simulink model "Copy_of_sliding_controller"  (R2021a)
settings: Solver=FixedStepAuto  StartTime=0.0  StopTime=inf  FixedStep=0.02  RelTol=1e-3
model workspace (MAT data in the model file):
  SL_ROS_VariableLengthArrays_MaxSizes.CommonInfo.ArrayTruncateAction = 'EmitWarning'
  SL_ROS_VariableLengthArrays_MaxSizes.MsgTypeMap = containers.Map
  SL_ROS_VariableLengthArrays_MaxSizes.MsgTypeMap.serialization.keys = {'ambf_walker/DesiredJoints', 'rbdl_server/RBDLInverseDynamicsRequest', 'rbdl_server/RBDLInverseDynamicsResponse', 'sensor_msgs/JointState'}
  SL_ROS_VariableLengthArrays_MaxSizes.MsgTypeMap.serialization.values{1}(1).PropertyName = 'Controller'
  SL_ROS_VariableLengthArrays_MaxSizes.MsgTypeMap.serialization.values{1}(1).DataType = 'uint8'
  SL_ROS_VariableLengthArrays_MaxSizes.MsgTypeMap.serialization.values{1}(1).MaxLength = 8
  SL_ROS_VariableLengthArrays_MaxSizes.MsgTypeMap.serialization.values{1}(2).PropertyName = 'Other'
  SL_ROS_VariableLengthArrays_MaxSizes.MsgTypeMap.serialization.values{1}(2).DataType = 'double'
  SL_ROS_VariableLengthArrays_MaxSizes.MsgTypeMap.serialization.values{1}(2).MaxLength = 7
  SL_ROS_VariableLengthArrays_MaxSizes.MsgTypeMap.serialization.values{1}(3).PropertyName = 'Q'
  SL_ROS_VariableLengthArrays_MaxSizes.MsgTypeMap.serialization.values{1}(3).DataType = 'double'
  SL_ROS_VariableLengthArrays_MaxSizes.MsgTypeMap.serialization.values{1}(3).MaxLength = 7
  SL_ROS_VariableLengthArrays_MaxSizes.MsgTypeMap.serialization.values{1}(4).PropertyName = 'Qd'
  SL_ROS_VariableLengthArrays_MaxSizes.MsgTypeMap.serialization.values{1}(4).DataType = 'double'
  SL_ROS_VariableLengthArrays_MaxSizes.MsgTypeMap.serialization.values{1}(4).MaxLength = 7
  SL_ROS_VariableLengthArrays_MaxSizes.MsgTypeMap.serialization.values{1}(5).PropertyName = 'Qdd'
  SL_ROS_VariableLengthArrays_MaxSizes.MsgTypeMap.serialization.values{1}(5).DataType = 'double'
  SL_ROS_VariableLengthArrays_MaxSizes.MsgTypeMap.serialization.values{1}(5).MaxLength = 7
  SL_ROS_VariableLengthArrays_MaxSizes.MsgTypeMap.serialization.values{2}(1).PropertyName = 'ModelName'
  SL_ROS_VariableLengthArrays_MaxSizes.MsgTypeMap.serialization.values{2}(1).DataType = 'uint8'
  SL_ROS_VariableLengthArrays_MaxSizes.MsgTypeMap.serialization.values{2}(1).MaxLength = 31
  SL_ROS_VariableLengthArrays_MaxSizes.MsgTypeMap.serialization.values{2}(2).PropertyName = 'Q'
  SL_ROS_VariableLengthArrays_MaxSizes.MsgTypeMap.serialization.values{2}(2).DataType = 'double'
  SL_ROS_VariableLengthArrays_MaxSizes.MsgTypeMap.serialization.values{2}(2).MaxLength = 7
  SL_ROS_VariableLengthArrays_MaxSizes.MsgTypeMap.serialization.values{2}(3).PropertyName = 'Qd'
  SL_ROS_VariableLengthArrays_MaxSizes.MsgTypeMap.serialization.values{2}(3).DataType = 'double'
  SL_ROS_VariableLengthArrays_MaxSizes.MsgTypeMap.serialization.values{2}(3).MaxLength = 7
  SL_ROS_VariableLengthArrays_MaxSizes.MsgTypeMap.serialization.values{2}(4).PropertyName = 'Qdd'
  SL_ROS_VariableLengthArrays_MaxSizes.MsgTypeMap.serialization.values{2}(4).DataType = 'double'
  SL_ROS_VariableLengthArrays_MaxSizes.MsgTypeMap.serialization.values{2}(4).MaxLength = 7
  SL_ROS_VariableLengthArrays_MaxSizes.MsgTypeMap.serialization.values{3}.PropertyName = 'Tau'
  SL_ROS_VariableLengthArrays_MaxSizes.MsgTypeMap.serialization.values{3}.DataType = 'double'
  SL_ROS_VariableLengthArrays_MaxSizes.MsgTypeMap.serialization.values{3}.MaxLength = 7
  SL_ROS_VariableLengthArrays_MaxSizes.MsgTypeMap.serialization.values{4}(1).PropertyName = 'Effort'
  SL_ROS_VariableLengthArrays_MaxSizes.MsgTypeMap.serialization.values{4}(1).DataType = 'double'
  SL_ROS_VariableLengthArrays_MaxSizes.MsgTypeMap.serialization.values{4}(1).MaxLength = 7
  SL_ROS_VariableLengthArrays_MaxSizes.MsgTypeMap.serialization.values{4}(2).PropertyName = 'Name'
  SL_ROS_VariableLengthArrays_MaxSizes.MsgTypeMap.serialization.values{4}(2).DataType = 'std_msgs/String'
  SL_ROS_VariableLengthArrays_MaxSizes.MsgTypeMap.serialization.values{4}(2).MaxLength = 16
  SL_ROS_VariableLengthArrays_MaxSizes.MsgTypeMap.serialization.values{4}(3).PropertyName = 'Position'
  SL_ROS_VariableLengthArrays_MaxSizes.MsgTypeMap.serialization.values{4}(3).DataType = 'double'
  SL_ROS_VariableLengthArrays_MaxSizes.MsgTypeMap.serialization.values{4}(3).MaxLength = 7
  SL_ROS_VariableLengthArrays_MaxSizes.MsgTypeMap.serialization.values{4}(4).PropertyName = 'Velocity'
  SL_ROS_VariableLengthArrays_MaxSizes.MsgTypeMap.serialization.values{4}(4).DataType = 'double'
  SL_ROS_VariableLengthArrays_MaxSizes.MsgTypeMap.serialization.values{4}(4).MaxLength = 7
  SL_ROS_VariableLengthArrays_MaxSizes.MsgTypeMap.serialization.uniformity = 0
  SL_ROS_VariableLengthArrays_MaxSizes.MsgTypeMap.serialization.keyType = 'char'
  SL_ROS_VariableLengthArrays_MaxSizes.MsgTypeMap.serialization.valueType = 'any'
values from neighbouring files (symbols this model uses):
  dampener = [30, 0; 0, 30]    [init_with_opt_gains.m]    (also in sliding_controller_init.m = 100*eye(2); trying01.m; trying02.m = [0.30, 0; 0, 0.30])
  Dm1 = [Dm_hip, 0.0, 0.0, 0.0, 0.0, 0.0,0 ... (first row only)    [init_with_opt_gains.m]    (also in sliding_controller_init.m = 30*eye(7); trying01.m; trying02.m = [101.7013888888889 0 0 0 0 0)
  exo_sat = 50    [init_with_opt_gains.m]    (also in sliding_controller_init.m; trying01.m = 250; trying02.m = 30)
  invMd = inv(Md)    [init_with_opt_gains.m]    (also in sliding_controller_init.m; trying01.m; trying02.m)
  Km1 = [Km_hip, 0.0, 0.0, 0.0, 0.0, 0.0,0 ... (first row only)    [init_with_opt_gains.m]    (also in sliding_controller_init.m = 30*eye(7); trying01.m; trying02.m = [6120.116528948097 0 0 0 0 0)
  l = [ 1.0, 1.5]    [sliding_controller_init.m]
  lambda2 = [lambda_hip, 0, 0, 0, 0, 0,0 ... (first row only)    [init_with_opt_gains.m]    (also in sliding_controller_init.m = eye(7); trying01.m; trying02.m = [lambda_hip, 0, 0, 0, 0, 0)
  mh = [2, 1]    [sliding_controller_init.m]
  rho2 = [rho_hip, 0.0, 0.0, 0.0, 0.0, 0.0,0 ... (first row only)    [init_with_opt_gains.m]    (also in sliding_controller_init.m = 200*eye(7); trying01.m; trying02.m = [rho_hip, 0.0, 0.0, 0.0, 0.0, 0.0)
  sat = 10    [sliding_controller_init.m]
  spring = [30, 0; 0, 30]    [init_with_opt_gains.m]    (also in sliding_controller_init.m = 100*eye(2); trying01.m; trying02.m = [0.30, 0; 0, 0.30])
undefined symbols (not defined in the file or in its folder): ModelName, Q, Qd, Qdd
libraries: robotlib x14
settings Model: Creator=nathanielgoldfarb  LastModifiedBy=nathanielgoldfarb
settings OptimizationCC: DefaultParameterBehavior=Inlined  EnhancedBackFolding=on  PassReuseOutputArgsAs=Individual arguments  ZeroExternalMemoryAtStartup=off  ZeroInternalMemoryAtStartup=off  InitFltsAndDblsToZero=on  MaxStackSize=64  OptimizeBlockOrder=speed  DifferentSizesBufferReuse=on  OptimizationCustomize=off  EfficientTunableParamExpr=on
settings DebuggingCC: ParameterTunabilityLossMsg=error
settings HardwareCC: TargetLongLongMode=on  UseEmbeddedCoderFeatures=off
settings SFSimCC: MATLABDynamicMemAlloc=off
settings RTWCC: SystemTargetFile=ert.tlc  TemplateMakefile=ert_default_tmf  Toolchain=Catkin
settings CodeAppCC: ForceParamTrailComments=on  IgnoreCustomStorageClasses=off  OperatorAnnotations=on  SimulinkDataObjDesc=on  SFDataObjDesc=on  InsertBlockDesc=on
settings ERTTargetCC: GenerateSampleERTMain=on  InlinedParameterPlacement=NonHierarchical  ERTCustomFileTemplate=example_file_process.tlc

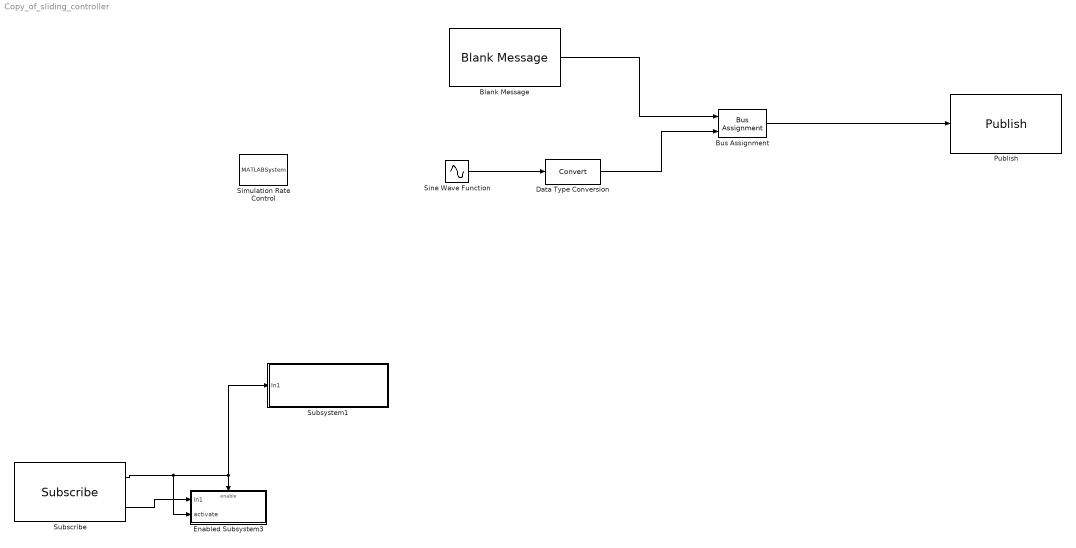
== system Copy_of_sliding_controller ==
  Blank Message : robotlib/Blank Message  messageClass=Message  entityType=std_msgs/Float32  messageType=std_msgs/Float32  SampleTime=-1  legacyBusStruct=off
  Bus Assignment : BusAssignment  AssignedSignals=Data
  Data Type Conversion : DataTypeConversion
  Enabled Subsystem3 : Subsystem  TreatAsAtomicUnit=on
  Publish : robotlib/Publish  topicSource=Specify your own  topic=/sin_wave  messageType=std_msgs/Float32  legacyBusStruct=off  messageQueueLength=1
  Simulation Rate Control : MATLABSystem  System=ExampleHelperSimulationRateControl  SampleTime=.02
      mask Type: ExampleHelperSimulationRateControl
      mask Display: disp('Rate Control');
  Sine Wave Function : Sin  SampleTime=0
  Subscribe : robotlib/Subscribe  topicSource=Select from ROS network  topic=/exosimulink_set_points  messageType=ambf_walker/DesiredJoints  SampleTime=-1  legacyBusStruct=off  messageQueueLength=1
  Subsystem1 : Subsystem
  wires:
  Subscribe/1 -> Enabled Subsystem3/2(activate), Subsystem1/1(In1), Enabled Subsystem3/Enable
  Data Type Conversion/1 -> Bus Assignment/2
  Blank Message/1 -> Bus Assignment/1
  Sine Wave Function/1 -> Data Type Conversion/1
  Bus Assignment/1 -> Publish/1
  Subscribe/2 -> Enabled Subsystem3/1(In1)

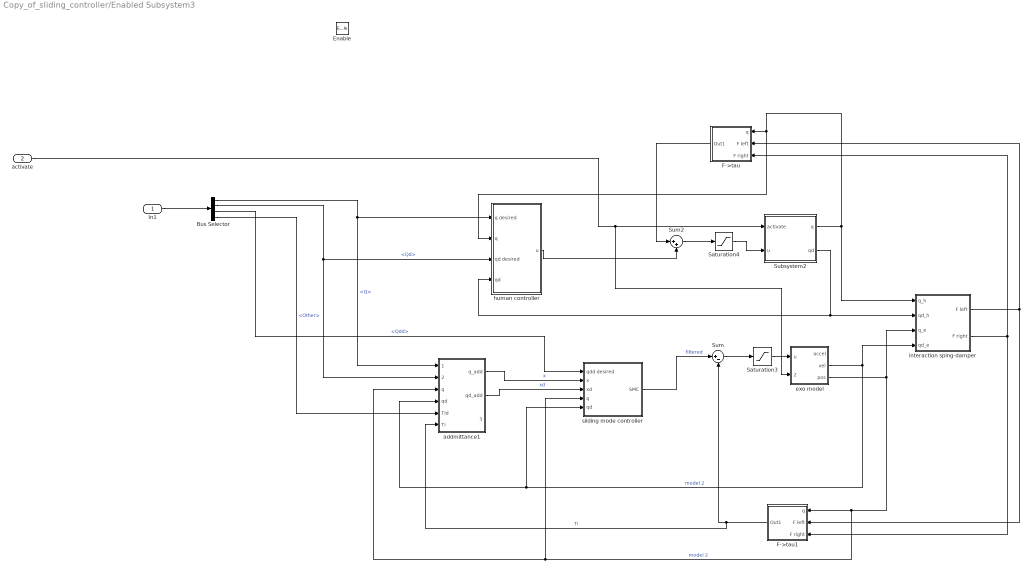
== system Copy_of_sliding_controller/Enabled Subsystem3 ==
  In1 : Inport
  activate : Inport  Port=2
  Enable : EnablePort
  " interaction sping-damper" : Subsystem
  Bus Selector : BusSelector  OutputSignals=Q,Qd,Qdd,Other
  F->tau : Subsystem
  F->tau1 : Subsystem
  Saturation3 : Saturate  UpperLimit=exo_sat  LowerLimit=-exo_sat
  Saturation4 : Saturate  UpperLimit=exo_sat  LowerLimit=-exo_sat
  Subsystem2 : Subsystem
  Sum : Sum  Inputs=|+-
  Sum2 : Sum  Inputs=|++
  addmittance1 : Subsystem
  exo model : Subsystem
  human controller : Subsystem
  sliding mode controller : Subsystem
  wires:
  exo model/3(pos) -> " interaction sping-damper"/3(q_e), addmittance1/3(q), sliding mode controller/4(q), F->tau1/1(q)  "model 2"
  Bus Selector/4 -> addmittance1/5(Tid)  "<Other>"
  Saturation3/1 -> exo model/1(u)
  addmittance1/2(qd_add) -> sliding mode controller/3(xd)  "xd"
  exo model/2(vel) -> " interaction sping-damper"/4("qd_e "), addmittance1/4(qd), sliding mode controller/5(qd)  "model 2"
  sliding mode controller/1(SMC) -> Sum/1  "filtered"
  " interaction sping-damper"/2(F right) -> F->tau1/3(F right), F->tau/3(F right)
  In1/1 -> Bus Selector/1
  human controller/1(u) -> Sum2/2
  Bus Selector/1 -> addmittance1/1(q desird), human controller/1(q desired)  "<Q>"
  Subsystem2/1(q) -> F->tau/1(q), human controller/2(q), " interaction sping-damper"/1(q_h)
  " interaction sping-damper"/1(F left) -> F->tau1/2(F left), F->tau/2(F left)
  Saturation4/1 -> Subsystem2/2(u)
  F->tau/1(Out1) -> Sum2/1
  addmittance1/1(q_add) -> sliding mode controller/2(x)  "x"
  Bus Selector/3 -> sliding mode controller/1(qdd desired)  "<Qdd>"
  Sum/1 -> Saturation3/1
  Bus Selector/2 -> addmittance1/2(qd desird), human controller/3(qd desired)  "<Qd>"
  Sum2/1 -> Saturation4/1
  Subsystem2/2(qd) -> human controller/4(qd), " interaction sping-damper"/2(qd_h)
  F->tau1/1(Out1) -> Sum/2, addmittance1/6(Ti)  "Ti"
  activate/1 -> exo model/2(activate), Subsystem2/1(activate)

== system Copy_of_sliding_controller/Subsystem1 ==
  In1 : Inport
  Constant : Constant  Value=false
  Data Type Conversion : DataTypeConversion
  If : If  IfExpression=u1 == 1
  If Action Subsystem : Subsystem  TreatAsAtomicUnit=on
  wires:
  In1/1 -> Data Type Conversion/1
  If/1 -> If Action Subsystem/Action
  Data Type Conversion/1 -> If/1
  Constant/1 -> If Action Subsystem/1(In1)

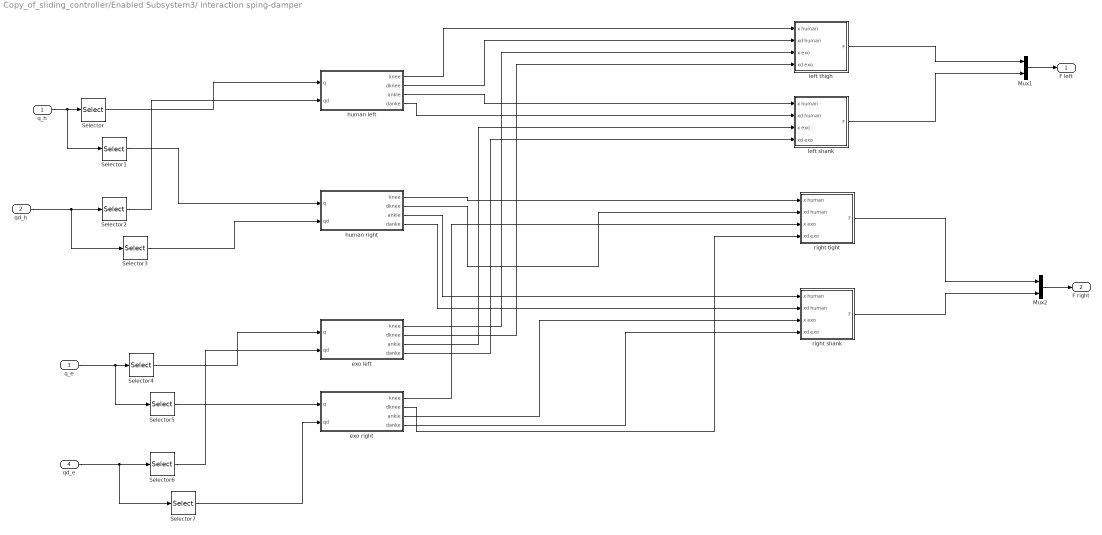
== system Copy_of_sliding_controller/Enabled Subsystem3/ interaction sping-damper ==
  q_h : Inport
  qd_h : Inport  Port=2
  q_e : Inport  Port=3
  "qd_e " : Inport  Port=4
  Mux1 : Mux  Inputs=2
  Mux2 : Mux  Inputs=2
  Selector{,2,4,6} (4 alike) : Selector  InputPortWidth=7  IndexOptions=Index vector (dialog)  Indices=[1 2]  OutputSizes=1
  Selector{1,3,5,7} (4 alike) : Selector  InputPortWidth=7  IndexOptions=Index vector (dialog)  Indices=[4 5]  OutputSizes=1
  exo left : MATLAB Function  TreatAsAtomicUnit=on
  exo right : MATLAB Function  TreatAsAtomicUnit=on
  human left : MATLAB Function  TreatAsAtomicUnit=on
  human right : MATLAB Function  TreatAsAtomicUnit=on
  left shank : Subsystem
  left thigh : Subsystem
  right shank : Subsystem
  right tight : Subsystem
  F left : Outport
  F right : Outport  Port=2
  wires:
  q_h/1 -> Selector1/1, Selector/1
  Selector/1 -> human left/1(q)
  Selector1/1 -> human right/1(q)
  Selector2/1 -> human left/2(qd)
  Selector3/1 -> human right/2(qd)
  qd_h/1 -> Selector3/1, Selector2/1
  q_e/1 -> Selector5/1, Selector4/1
  Selector4/1 -> exo left/1(q)
  Selector5/1 -> exo right/1(q)
  "qd_e "/1 -> Selector7/1, Selector6/1
  Selector7/1 -> exo right/2(qd)
  Selector6/1 -> exo left/2(qd)
  human left/1(knee) -> left thigh/1(x human)
  human left/2(dknee) -> left thigh/2("xd human ")
  human left/3(ankle) -> left shank/1(x human)
  human left/4(danke) -> left shank/2("xd human ")
  exo left/1(knee) -> left thigh/3(x exo)
  exo left/2(dknee) -> left thigh/4(xd exo)
  exo left/3(ankle) -> left shank/3(x exo)
  exo left/4(danke) -> left shank/4(xd exo)
  human right/4(danke) -> right shank/2("xd human ")
  exo right/1(knee) -> right tight/3(x exo)
  human right/1(knee) -> right tight/1(x human)
  exo right/3(ankle) -> right shank/3(x exo)
  exo right/4(danke) -> right shank/4(xd exo)
  exo right/2(dknee) -> right tight/4(xd exo)
  human right/3(ankle) -> right shank/1(x human)
  human right/2(dknee) -> right tight/2("xd human ")
  Mux1/1 -> F left/1
  left shank/1(F) -> Mux1/2
  left thigh/1(F) -> Mux1/1
  Mux2/1 -> F right/1
  right tight/1(F) -> Mux2/1
  right shank/1(F) -> Mux2/2

== system Copy_of_sliding_controller/Enabled Subsystem3/F->tau ==
  q : Inport
  F left : Inport  Port=2
  F right : Inport  Port=3
  Constant : Constant  Value=0
  Mux : Mux  Inputs=3
  Selector : Selector  InputPortWidth=7  IndexOptions=Index vector (dialog)  Indices=[1 2]  OutputSizes=1
  Selector1 : Selector  InputPortWidth=7  IndexOptions=Index vector (dialog)  Indices=[4 5]  OutputSizes=1
  Subsystem : Subsystem
  Subsystem2 : Subsystem
  Out1 : Outport
  wires:
  Subsystem/1(tau) -> Mux/1
  q/1 -> Selector1/1, Selector/1
  Selector/1 -> Subsystem/1(q)
  F left/1 -> Subsystem/2(F)
  Selector1/1 -> Subsystem2/1(q)
  F right/1 -> Subsystem2/2(F)
  Subsystem2/1(tau) -> Mux/2
  Mux/1 -> Out1/1
  Constant/1 -> Mux/3

== system Copy_of_sliding_controller/Enabled Subsystem3/F->tau1 ==
  q : Inport
  F left : Inport  Port=2
  F right : Inport  Port=3
  Constant : Constant  Value=0
  Mux : Mux  Inputs=3
  Selector : Selector  InputPortWidth=7  IndexOptions=Index vector (dialog)  Indices=[1 2]  OutputSizes=1
  Selector1 : Selector  InputPortWidth=7  IndexOptions=Index vector (dialog)  Indices=[4 5]  OutputSizes=1
  Subsystem : Subsystem
  Subsystem2 : Subsystem
  Out1 : Outport
  wires:
  Subsystem/1(tau) -> Mux/1
  q/1 -> Selector1/1, Selector/1
  Selector/1 -> Subsystem/1(q)
  F left/1 -> Subsystem/2(F)
  Selector1/1 -> Subsystem2/1(q)
  F right/1 -> Subsystem2/2(F)
  Subsystem2/1(tau) -> Mux/2
  Mux/1 -> Out1/1
  Constant/1 -> Mux/3

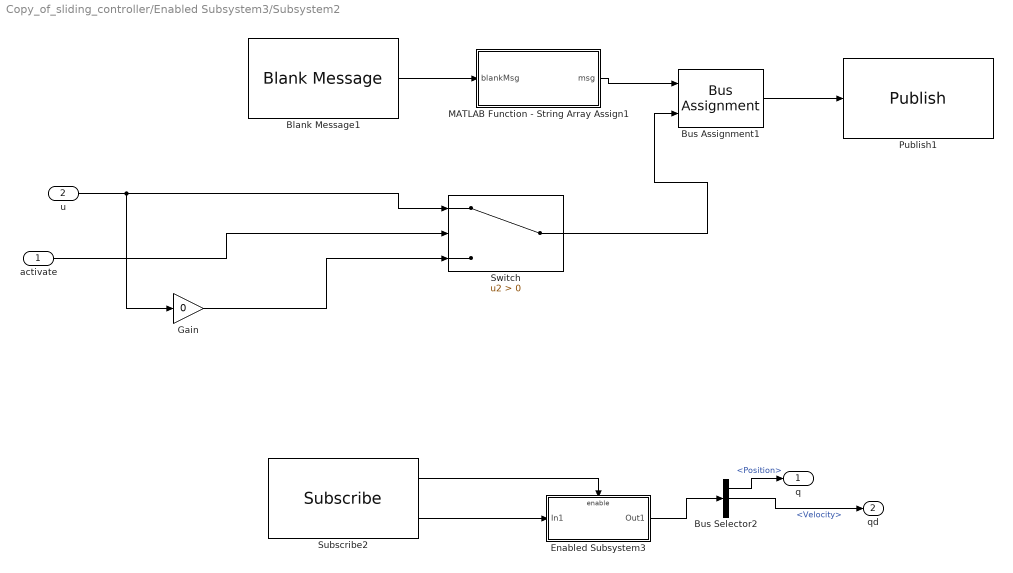
== system Copy_of_sliding_controller/Enabled Subsystem3/Subsystem2 ==
  activate : Inport
  u : Inport  Port=2
  Blank Message1 : robotlib/Blank Message  messageClass=Message  entityType=sensor_msgs/JointState  messageType=sensor_msgs/JointState  SampleTime=inf  legacyBusStruct=off
  Bus Assignment1 : BusAssignment  AssignedSignals=Effort
  Bus Selector2 : BusSelector  OutputSignals=Position,Velocity,Effort
  Enabled Subsystem3 : Subsystem  TreatAsAtomicUnit=on
  Gain : Gain  Gain=0
  MATLAB Function - String Array Assign1 : MATLAB Function  TreatAsAtomicUnit=on
  Publish1 : robotlib/Publish  topicSource=Specify your own  topic=/human_simulink_jointstate  messageType=sensor_msgs/JointState  legacyBusStruct=off  messageQueueLength=1
  Subscribe2 : robotlib/Subscribe  topicSource=Select from ROS network  topic=/human_jointstate  messageType=sensor_msgs/JointState  SampleTime=-1  legacyBusStruct=off  messageQueueLength=1
  Switch : Switch  Criteria=u2 > Threshold
  q : Outport
  qd : Outport  Port=2
  wires:
  Subscribe2/2 -> Enabled Subsystem3/1(In1)
  Enabled Subsystem3/1(Out1) -> Bus Selector2/1
  Bus Assignment1/1 -> Publish1/1
  MATLAB Function - String Array Assign1/1(msg) -> Bus Assignment1/1
  Bus Selector2/2 -> qd/1  "<Velocity>"
  Blank Message1/1 -> MATLAB Function - String Array Assign1/1(blankMsg)
  Subscribe2/1 -> Enabled Subsystem3/Enable
  Bus Selector2/1 -> q/1  "<Position>"
  Gain/1 -> Switch/3
  Switch/1 -> Bus Assignment1/2
  u/1 -> Gain/1, Switch/1
  activate/1 -> Switch/2

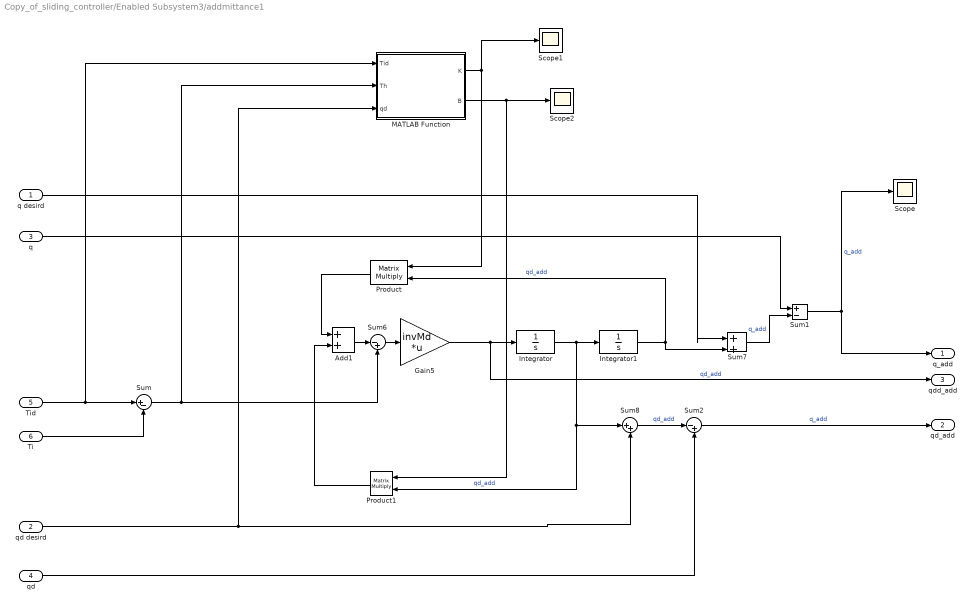
== system Copy_of_sliding_controller/Enabled Subsystem3/addmittance1 ==
  q desird : Inport
  qd desird : Inport  Port=2
  q : Inport  Port=3
  qd : Inport  Port=4
  Tid : Inport  Port=5
  Ti : Inport  Port=6
  Add1 : Sum
  Gain5 : Gain  Gain=invMd  Multiplication=Matrix(K*u)
  Integrator : Integrator
  Integrator1 : Integrator  InitialCondition=[-0.349,-0.2,0,-0.349,-0.2,0,0]
  MATLAB Function : MATLAB Function  TreatAsAtomicUnit=on
  Product : Product  Multiplication=Matrix(*)
  Product1 : Product  Multiplication=Matrix(*)
  Scope : Scope
  Scope1 : Scope
  Scope2 : Scope
  Sum : Sum  Inputs=|+-
  Sum1 : Sum  Inputs=|+-
  Sum2 : Sum  Inputs=|-+
  Sum6 : Sum  Inputs=|-+
  Sum7 : Sum  Inputs=|++
  Sum8 : Sum  Inputs=|++
  q_add : Outport
  qd_add : Outport  Port=2
  qdd_add : Outport  Port=3
  wires:
  Add1/1 -> Sum6/1
  qd desird/1 -> MATLAB Function/3(qd), Sum8/2
  Gain5/1 -> qdd_add/1, Integrator/1  "qd_add"
  Sum6/1 -> Gain5/1
  Product/1 -> Add1/1
  q desird/1 -> Sum7/1
  qd/1 -> Sum2/2
  Sum2/1 -> qd_add/1  "q_add"
  Sum7/1 -> Sum1/2  "q_add"
  q/1 -> Sum1/1
  Sum1/1 -> q_add/1, Scope/1  "q_add"
  Sum8/1 -> Sum2/1  "qd_add"
  Integrator/1 -> Product1/2, Sum8/1, Integrator1/1  "qd_add"
  Integrator1/1 -> Product/2, Sum7/2  "qd_add"
  Sum/1 -> MATLAB Function/2(Th), Sum6/2
  Tid/1 -> MATLAB Function/1(Tid), Sum/1
  Ti/1 -> Sum/2
  Product1/1 -> Add1/2
  MATLAB Function/1(K) -> Scope1/1, Product/1
  MATLAB Function/2(B) -> Scope2/1, Product1/1

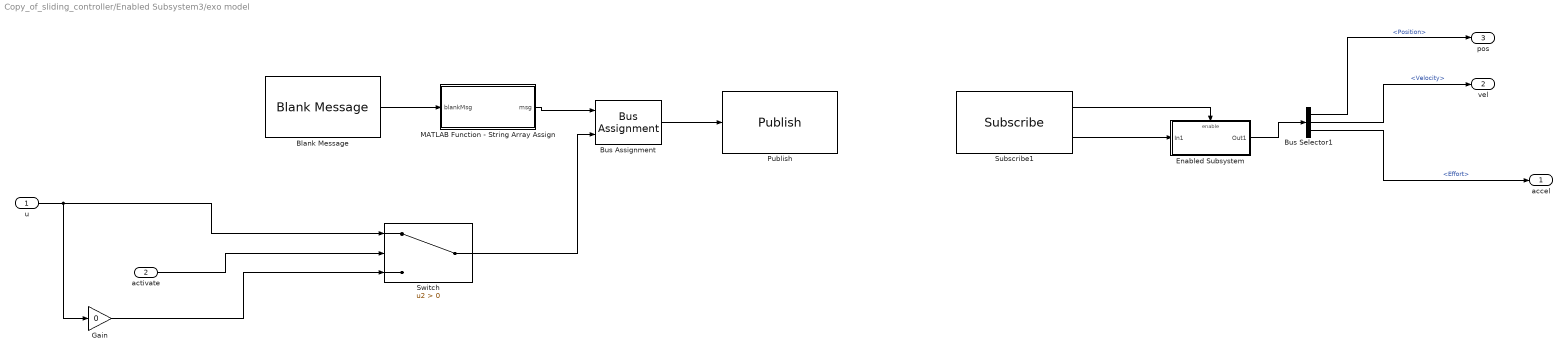
== system Copy_of_sliding_controller/Enabled Subsystem3/exo model ==
  u : Inport
  activate : Inport  Port=2
  Blank Message : robotlib/Blank Message  messageClass=Message  entityType=sensor_msgs/JointState  messageType=sensor_msgs/JointState  SampleTime=inf  legacyBusStruct=off
  Bus Assignment : BusAssignment  AssignedSignals=Effort
  Bus Selector1 : BusSelector  OutputSignals=Position,Velocity,Effort
  Enabled Subsystem : Subsystem  TreatAsAtomicUnit=on
  Gain : Gain  Gain=0
  MATLAB Function - String Array Assign : MATLAB Function  TreatAsAtomicUnit=on
  Publish : robotlib/Publish  topicSource=Specify your own  topic=/exo_simulink_jointstate  messageType=sensor_msgs/JointState  legacyBusStruct=off  messageQueueLength=1
  Subscribe1 : robotlib/Subscribe  topicSource=Select from ROS network  topic=/exo_jointstate  messageType=sensor_msgs/JointState  SampleTime=-1  legacyBusStruct=off  messageQueueLength=1
  Switch : Switch  Criteria=u2 > Threshold
  accel : Outport
  vel : Outport  Port=2
  pos : Outport  Port=3
  wires:
  Subscribe1/1 -> Enabled Subsystem/Enable
  Bus Selector1/1 -> pos/1  "<Position>"
  Enabled Subsystem/1(Out1) -> Bus Selector1/1
  Subscribe1/2 -> Enabled Subsystem/1(In1)
  Bus Selector1/2 -> vel/1  "<Velocity>"
  Bus Assignment/1 -> Publish/1
  MATLAB Function - String Array Assign/1(msg) -> Bus Assignment/1
  Bus Selector1/3 -> accel/1  "<Effort>"
  Blank Message/1 -> MATLAB Function - String Array Assign/1(blankMsg)
  Gain/1 -> Switch/3
  activate/1 -> Switch/2
  Switch/1 -> Bus Assignment/2
  u/1 -> Gain/1, Switch/1

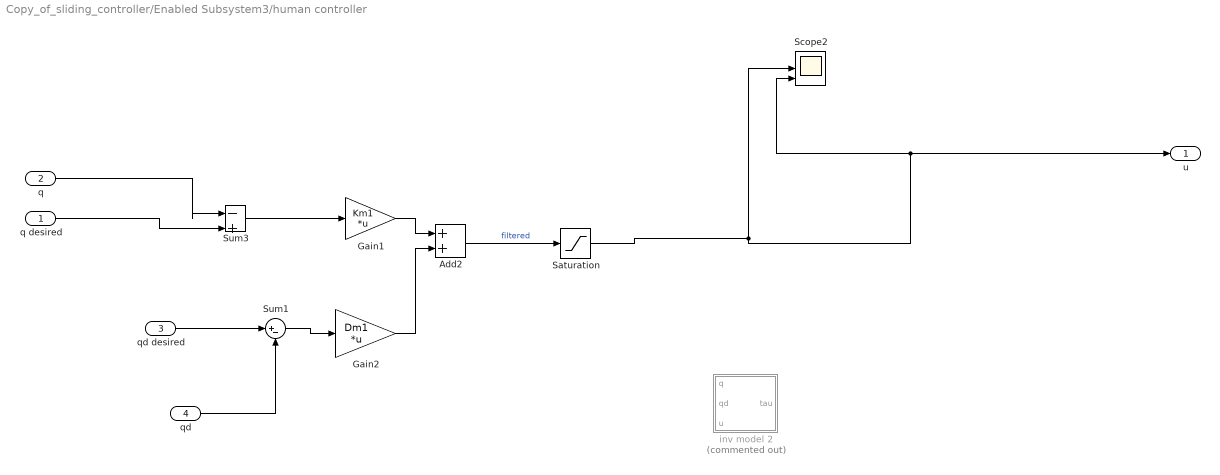
== system Copy_of_sliding_controller/Enabled Subsystem3/human controller ==
  q desired : Inport
  q : Inport  Port=2
  qd desired : Inport  Port=3
  qd : Inport  Port=4
  Add2 : Sum
  Gain1 : Gain  Gain=Km1  Multiplication=Matrix(K*u)
  Gain2 : Gain  Gain=Dm1  Multiplication=Matrix(K*u)
  Saturation : Saturate  UpperLimit=sat  LowerLimit=-sat
  Scope2 : Scope  NumInputPorts=3
  Sum1 : Sum  Inputs=|+-
  Sum3 : Sum  Inputs=|-+
  inv model 2 : Subsystem  Commented=on
  u : Outport
  wires:
  Sum1/1 -> Gain2/1
  qd/1 -> Sum1/2
  Sum3/1 -> Gain1/1
  Gain2/1 -> Add2/2
  q desired/1 -> Sum3/2
  Gain1/1 -> Add2/1
  qd desired/1 -> Sum1/1
  q/1 -> Sum3/1
  Add2/1 -> Saturation/1  "filtered"
  Saturation/1 -> u/1, Scope2/3, Scope2/2

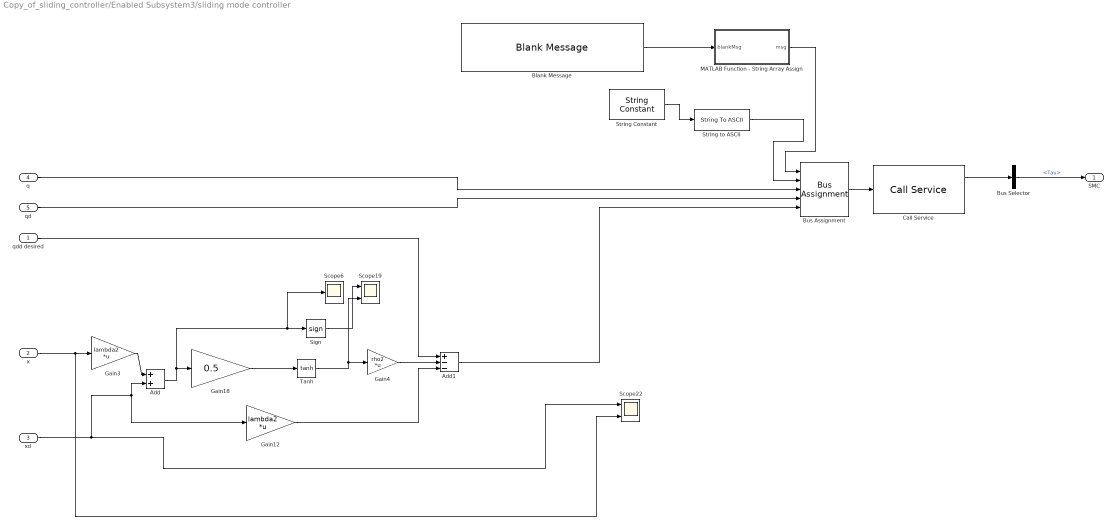
== system Copy_of_sliding_controller/Enabled Subsystem3/sliding mode controller ==
  qdd desired : Inport
  x : Inport  Port=2
  xd : Inport  Port=3
  q : Inport  Port=4
  qd : Inport  Port=5
  Add : Sum
  Add1 : Sum  Inputs=+--
  Blank Message : robotlib/Blank Message  messageClass=Service Request  entityType=rbdl_server/RBDLInverseDynamics  messageType=rbdl_server/RBDLInverseDynamicsRequest  SampleTime=inf  legacyBusStruct=off
  Bus Assignment : BusAssignment  AssignedSignals=ModelName,Q,Qd,Qdd
  Bus Selector : BusSelector  OutputSignals=Tau
  Call Service : robotlib/Call Service  topicSource=Select from ROS network  service=/InverseDynamics  serviceType=rbdl_server/RBDLInverseDynamics  connectionTimeout=5  keepPersistent=off  ShowErrorCodeOutput=on  legacyBusStruct=off
      settings: SourceProductBaseCode=RR
  Gain12 : Gain  Gain=lambda2  Multiplication=Matrix(K*u)
  Gain18 : Gain  Gain=0.5
  Gain3 : Gain  Gain=lambda2  Multiplication=Matrix(K*u)
  Gain4 : Gain  Gain=rho2  Multiplication=Matrix(K*u)
  MATLAB Function - String Array Assign : MATLAB Function  TreatAsAtomicUnit=on
  Scope19 : Scope  NumInputPorts=2
  Scope22 : Scope  NumInputPorts=2
  Scope6 : Scope
  Sign : Signum
  String Constant : StringConstant  String='exo'
  String to ASCII : StringToASCII
  Tanh : Trigonometry  Operator=tanh
  SMC : Outport
  wires:
  Gain18/1 -> Tanh/1
  Gain12/1 -> Add1/3
  Gain3/1 -> Add/1
  x/1 -> Scope22/2, Gain3/1
  xd/1 -> Add/2, Gain12/1, Scope22/1
  Add/1 -> Scope6/1, Sign/1, Gain18/1
  Add1/1 -> Bus Assignment/5
  Sign/1 -> Scope19/1
  Gain4/1 -> Add1/2
  qdd desired/1 -> Add1/1
  Tanh/1 -> Gain4/1, Scope19/2
  q/1 -> Bus Assignment/3
  qd/1 -> Bus Assignment/4
  Blank Message/1 -> MATLAB Function - String Array Assign/1(blankMsg)
  MATLAB Function - String Array Assign/1(msg) -> Bus Assignment/1
  Bus Assignment/1 -> Call Service/1
  Call Service/1 -> Bus Selector/1
  String Constant/1 -> String to ASCII/1
  String to ASCII/1 -> Bus Assignment/2
  Bus Selector/1 -> SMC/1  "<Tau>"

== system Copy_of_sliding_controller/Subsystem1/If Action Subsystem ==
  In1 : Inport
  Action Port : ActionPort  ActionPortLabel=if(u1 == 1)
  Blank Message : robotlib/Blank Message  messageClass=Service Request  entityType=std_srvs/SetBool  messageType=std_srvs/SetBoolRequest  SampleTime=inf  legacyBusStruct=off
  Bus Assignment : BusAssignment  AssignedSignals=Data
  Bus Assignment1 : BusAssignment  AssignedSignals=Data
  Call Service : robotlib/Call Service  topicSource=Select from ROS network  service=/exo_controller_onoff  serviceType=std_srvs/SetBool  connectionTimeout=5  keepPersistent=on  ShowErrorCodeOutput=on  legacyBusStruct=off
      settings: SourceProductBaseCode=RR
  Call Service1 : robotlib/Call Service  topicSource=Select from ROS network  service=/human_controller_onoff  serviceType=std_srvs/SetBool  connectionTimeout=5  keepPersistent=on  ShowErrorCodeOutput=on  legacyBusStruct=off
      settings: SourceProductBaseCode=RR
  Terminator1 : Terminator
  Terminator2 : Terminator
  exo internal controller state : Outport
  human internal controller state1 : Outport  Port=2
  wires:
  In1/1 -> Bus Assignment/2, Bus Assignment1/2
  Bus Assignment1/1 -> Call Service1/1
  Call Service/1 -> exo internal controller state/1
  Bus Assignment/1 -> Call Service/1
  Call Service/2 -> Terminator2/1
  Blank Message/1 -> Bus Assignment1/1, Bus Assignment/1
  Call Service1/1 -> human internal controller state1/1
  Call Service1/2 -> Terminator1/1

== system Copy_of_sliding_controller/Enabled Subsystem3/ interaction sping-damper/left shank ==
  x human : Inport
  "xd human " : Inport  Port=2
  x exo : Inport  Port=3
  xd exo : Inport  Port=4
  Gain3 : Gain  Gain=spring  Multiplication=Matrix(K*u)
  Gain4 : Gain  Gain=dampener  Multiplication=Matrix(K*u)
  Subtract : Sum  Inputs=-+
  Subtract1 : Sum  Inputs=-+
  Subtract2 : Sum
  F : Outport
  wires:
  Subtract2/1 -> F/1
  xd exo/1 -> Subtract1/2
  Gain4/1 -> Subtract2/2
  Subtract/1 -> Gain3/1
  Subtract1/1 -> Gain4/1
  x exo/1 -> Subtract/2
  x human/1 -> Subtract/1
  "xd human "/1 -> Subtract1/1
  Gain3/1 -> Subtract2/1

== system Copy_of_sliding_controller/Enabled Subsystem3/ interaction sping-damper/left thigh ==
  x human : Inport
  "xd human " : Inport  Port=2
  x exo : Inport  Port=3
  xd exo : Inport  Port=4
  Gain3 : Gain  Gain=spring  Multiplication=Matrix(K*u)
  Gain4 : Gain  Gain=dampener  Multiplication=Matrix(K*u)
  Subtract : Sum  Inputs=-+
  Subtract1 : Sum  Inputs=-+
  Subtract2 : Sum
  F : Outport
  wires:
  Subtract2/1 -> F/1
  xd exo/1 -> Subtract1/2
  Gain4/1 -> Subtract2/2
  Subtract/1 -> Gain3/1
  Subtract1/1 -> Gain4/1
  x exo/1 -> Subtract/2
  x human/1 -> Subtract/1
  "xd human "/1 -> Subtract1/1
  Gain3/1 -> Subtract2/1

== system Copy_of_sliding_controller/Enabled Subsystem3/ interaction sping-damper/right shank ==
  x human : Inport
  "xd human " : Inport  Port=2
  x exo : Inport  Port=3
  xd exo : Inport  Port=4
  Gain3 : Gain  Gain=spring  Multiplication=Matrix(K*u)
  Gain4 : Gain  Gain=dampener  Multiplication=Matrix(K*u)
  Subtract : Sum  Inputs=-+
  Subtract1 : Sum  Inputs=-+
  Subtract2 : Sum
  F : Outport
  wires:
  Subtract2/1 -> F/1
  xd exo/1 -> Subtract1/2
  Gain4/1 -> Subtract2/2
  Subtract/1 -> Gain3/1
  Subtract1/1 -> Gain4/1
  x exo/1 -> Subtract/2
  x human/1 -> Subtract/1
  "xd human "/1 -> Subtract1/1
  Gain3/1 -> Subtract2/1

== system Copy_of_sliding_controller/Enabled Subsystem3/ interaction sping-damper/right tight ==
  x human : Inport
  "xd human " : Inport  Port=2
  x exo : Inport  Port=3
  xd exo : Inport  Port=4
  Gain3 : Gain  Gain=spring  Multiplication=Matrix(K*u)
  Gain4 : Gain  Gain=dampener  Multiplication=Matrix(K*u)
  Subtract : Sum  Inputs=-+
  Subtract1 : Sum  Inputs=-+
  Subtract2 : Sum
  F : Outport
  wires:
  Subtract2/1 -> F/1
  xd exo/1 -> Subtract1/2
  Gain4/1 -> Subtract2/2
  Subtract/1 -> Gain3/1
  Subtract1/1 -> Gain4/1
  x exo/1 -> Subtract/2
  x human/1 -> Subtract/1
  "xd human "/1 -> Subtract1/1
  Gain3/1 -> Subtract2/1

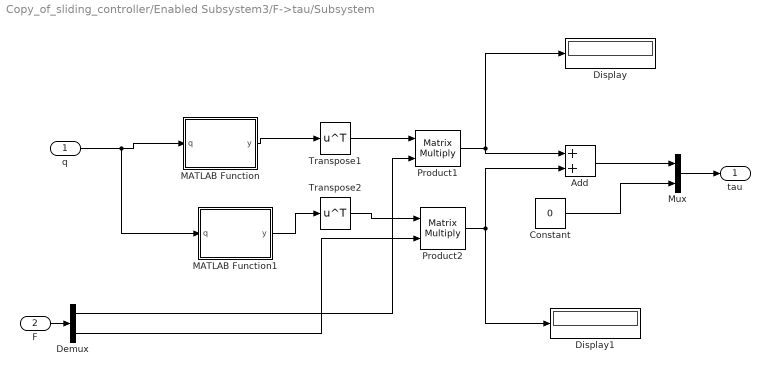
== system Copy_of_sliding_controller/Enabled Subsystem3/F->tau/Subsystem ==
  q : Inport
  F : Inport  Port=2
  Add : Sum
  Constant : Constant  Value=0
  Demux : Demux  Outputs=2
  Display : Display
  Display1 : Display
  MATLAB Function : MATLAB Function  TreatAsAtomicUnit=on
  MATLAB Function1 : MATLAB Function  TreatAsAtomicUnit=on
  Mux : Mux  Inputs=2
  Product1 : Product  Multiplication=Matrix(*)
  Product2 : Product  Multiplication=Matrix(*)
  Transpose1 : Math  Operator=transpose  SaturateOnIntegerOverflow=on
  Transpose2 : Math  Operator=transpose  SaturateOnIntegerOverflow=on
  tau : Outport
  wires:
  MATLAB Function1/1(y) -> Transpose2/1
  Transpose2/1 -> Product2/1
  Product1/1 -> Add/1, Display/1
  F/1 -> Demux/1
  Product2/1 -> Add/2, Display1/1
  Transpose1/1 -> Product1/1
  MATLAB Function/1(y) -> Transpose1/1
  q/1 -> MATLAB Function1/1(q), MATLAB Function/1(q)
  Demux/2 -> Product2/2
  Demux/1 -> Product1/2
  Mux/1 -> tau/1
  Add/1 -> Mux/1
  Constant/1 -> Mux/2

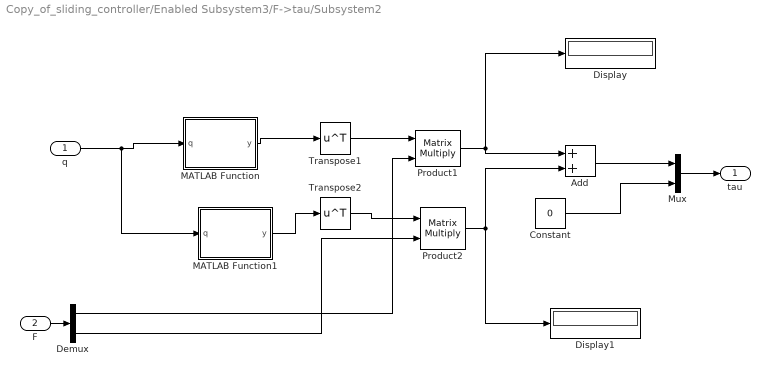
== system Copy_of_sliding_controller/Enabled Subsystem3/F->tau/Subsystem2 ==
  q : Inport
  F : Inport  Port=2
  Add : Sum
  Constant : Constant  Value=0
  Demux : Demux  Outputs=2
  Display : Display
  Display1 : Display
  MATLAB Function : MATLAB Function  TreatAsAtomicUnit=on
  MATLAB Function1 : MATLAB Function  TreatAsAtomicUnit=on
  Mux : Mux  Inputs=2
  Product1 : Product  Multiplication=Matrix(*)
  Product2 : Product  Multiplication=Matrix(*)
  Transpose1 : Math  Operator=transpose  SaturateOnIntegerOverflow=on
  Transpose2 : Math  Operator=transpose  SaturateOnIntegerOverflow=on
  tau : Outport
  wires:
  MATLAB Function1/1(y) -> Transpose2/1
  Transpose2/1 -> Product2/1
  Product1/1 -> Add/1, Display/1
  F/1 -> Demux/1
  Product2/1 -> Add/2, Display1/1
  Transpose1/1 -> Product1/1
  MATLAB Function/1(y) -> Transpose1/1
  q/1 -> MATLAB Function1/1(q), MATLAB Function/1(q)
  Demux/2 -> Product2/2
  Demux/1 -> Product1/2
  Mux/1 -> tau/1
  Add/1 -> Mux/1
  Constant/1 -> Mux/2

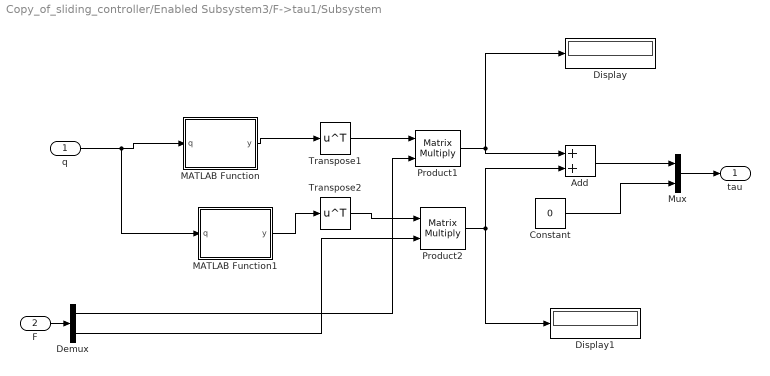
== system Copy_of_sliding_controller/Enabled Subsystem3/F->tau1/Subsystem ==
  q : Inport
  F : Inport  Port=2
  Add : Sum
  Constant : Constant  Value=0
  Demux : Demux  Outputs=2
  Display : Display
  Display1 : Display
  MATLAB Function : MATLAB Function  TreatAsAtomicUnit=on
  MATLAB Function1 : MATLAB Function  TreatAsAtomicUnit=on
  Mux : Mux  Inputs=2
  Product1 : Product  Multiplication=Matrix(*)
  Product2 : Product  Multiplication=Matrix(*)
  Transpose1 : Math  Operator=transpose  SaturateOnIntegerOverflow=on
  Transpose2 : Math  Operator=transpose  SaturateOnIntegerOverflow=on
  tau : Outport
  wires:
  MATLAB Function1/1(y) -> Transpose2/1
  Transpose2/1 -> Product2/1
  Product1/1 -> Add/1, Display/1
  F/1 -> Demux/1
  Product2/1 -> Add/2, Display1/1
  Transpose1/1 -> Product1/1
  MATLAB Function/1(y) -> Transpose1/1
  q/1 -> MATLAB Function1/1(q), MATLAB Function/1(q)
  Demux/2 -> Product2/2
  Demux/1 -> Product1/2
  Mux/1 -> tau/1
  Add/1 -> Mux/1
  Constant/1 -> Mux/2

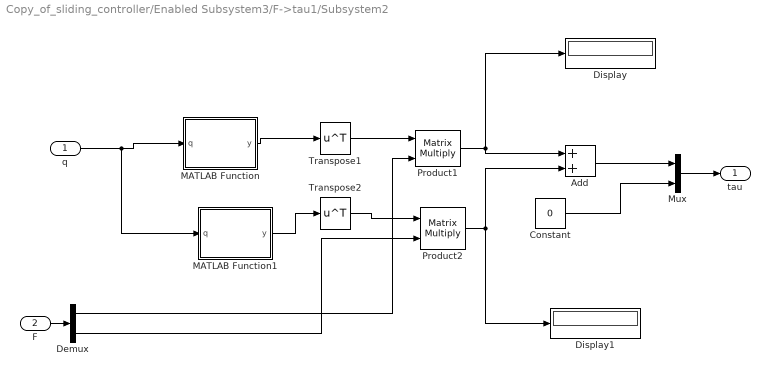
== system Copy_of_sliding_controller/Enabled Subsystem3/F->tau1/Subsystem2 ==
  q : Inport
  F : Inport  Port=2
  Add : Sum
  Constant : Constant  Value=0
  Demux : Demux  Outputs=2
  Display : Display
  Display1 : Display
  MATLAB Function : MATLAB Function  TreatAsAtomicUnit=on
  MATLAB Function1 : MATLAB Function  TreatAsAtomicUnit=on
  Mux : Mux  Inputs=2
  Product1 : Product  Multiplication=Matrix(*)
  Product2 : Product  Multiplication=Matrix(*)
  Transpose1 : Math  Operator=transpose  SaturateOnIntegerOverflow=on
  Transpose2 : Math  Operator=transpose  SaturateOnIntegerOverflow=on
  tau : Outport
  wires:
  MATLAB Function1/1(y) -> Transpose2/1
  Transpose2/1 -> Product2/1
  Product1/1 -> Add/1, Display/1
  F/1 -> Demux/1
  Product2/1 -> Add/2, Display1/1
  Transpose1/1 -> Product1/1
  MATLAB Function/1(y) -> Transpose1/1
  q/1 -> MATLAB Function1/1(q), MATLAB Function/1(q)
  Demux/2 -> Product2/2
  Demux/1 -> Product1/2
  Mux/1 -> tau/1
  Add/1 -> Mux/1
  Constant/1 -> Mux/2

== system Copy_of_sliding_controller/Enabled Subsystem3/Subsystem2/Enabled Subsystem3 ==
  In1 : Inport
  Enable : EnablePort
  Out1 : Outport
  wires:
  In1/1 -> Out1/1

== system Copy_of_sliding_controller/Enabled Subsystem3/exo model/Enabled Subsystem ==
  In1 : Inport
  Enable : EnablePort
  Out1 : Outport
  wires:
  In1/1 -> Out1/1

== system Copy_of_sliding_controller/Enabled Subsystem3/human controller/inv model 2 ==
  q : Inport
  qd : Inport  Port=2
  "u " : Inport  Port=3
  Add2 : Sum  Inputs=+++
  C : MATLAB Function  TreatAsAtomicUnit=on
  Constant : Constant  Value=mh
  Constant1 : Constant  Value=l
  G : MATLAB Function  TreatAsAtomicUnit=on
  M : MATLAB Function  TreatAsAtomicUnit=on
  Product : Product  Multiplication=Matrix(*)
  "tau " : Outport
  wires:
  Constant1/1 -> C/2(l), M/2(l)
  Constant/1 -> G/1(m), C/1(m), M/1(m)
  "u "/1 -> Product/2
  Product/1 -> Add2/1
  M/1(y) -> Product/1
  qd/1 -> C/4(qd)
  q/1 -> G/2(q), C/3(q), M/3(q)
  Add2/1 -> "tau "/1
  C/1(y) -> Add2/2
  G/1(y) -> Add2/3

== matlab function Copy_of_sliding_controller/Enabled Subsystem3/Subsystem2/MATLAB Function - String Array Assign1 ==
  data: blankMsg input; msg output Bus: SL_Bus_sliding_controller_sensor_msgs_JointState
function msg = stringArrayAssign(blankMsg)
% stringArrayAssign - Assign a string array in a ROS message
%
%  blankMsg (input): A bus for a 'sensor_msgs/JointState' message. This is 
%      used to initialize the output.
%  msg (output): A bus for a 'sensor_msgs/JointState' message message, with 
%      Name field set to a string array.
%
%   Copyright 2015 The MathWorks, Inc.

%#codegen

% Note: The datatype of 'msg' has been explicitly set to the appropriate 
% Simulink bus type ("SL_Bus_robotROSMessageUsageExample_sensor_msgs_JointState"). 
%
% If the model name is changed, the datatype needs to be changed as well:
%   1) Click "Edit Data" in the Editor toolstrip to open "Ports and Data Manager"
%   2) Select "msg". From the "Type" dropdown, select "--- Refresh data types ---"
%   3) Set datatype to "Bus: SL_Bus_<modelname>_sensor_msgs_JointState"

strArrayToAssign = {'LeftHumanHip', 'LeftHumanKnee', 'LeftHumanAnkle', 'RightHumanHip', 'RightHumanKnee', 'RightHumanAnkle'};
msg = blankMsg;

% Set the number of strings in the string array.
% msg (sensor_msgs/JointState) includes the following fields
%           Name : array of std_msgs/String (string array)
%   Name_SL_Info : struct with fields CurrentLength, ReceivedLength
numStringsInArray = length(strArrayToAssign);
msg.Name_SL_Info.CurrentLength = uint32(numStringsInArray);
msg.Effort_SL_Info.CurrentLength = uint32(numStringsInArray);

% Set the individual strings in the array
for idx=1:numStringsInArray
    str = strArrayToAssign{idx};
    strLength = length(str);
    msg.Name(idx).Data(1:strLength) = uint8(str);
    msg.Name(idx).Data_SL_Info.CurrentLength = uint32(strLength);
end

== matlab function Copy_of_sliding_controller/Enabled Subsystem3/ interaction sping-damper/exo left ==
  data: q input; knee output; dknee output; qd input; ankle output; danke output
function [knee, dknee,ankle, danke]  = fcn(q, qd)


[knee, ankle, dknee, danke] = forward_kinimatics_leg(q,qd);
end

== matlab function Copy_of_sliding_controller/Enabled Subsystem3/ interaction sping-damper/exo right ==
  data: q input; knee output; dknee output; qd input; ankle output; danke output
function [knee, dknee,ankle, danke]  = fcn(q, qd)


[knee, ankle, dknee, danke] = forward_kinimatics_leg(q,qd);
end

== matlab function Copy_of_sliding_controller/Enabled Subsystem3/F->tau1/Subsystem/MATLAB Function ==
  data: q input; y output
function y = fcn(q)

l1 = 0.3240;
y = [-l1*sin(q(1)), 0; l1*cos(q(1)), 0 ];


end

== matlab function Copy_of_sliding_controller/Enabled Subsystem3/ interaction sping-damper/human left ==
  data: q input; knee output; dknee output; qd input; ankle output; danke output
function [knee, dknee,ankle, danke]  = fcn(q, qd)


[knee, ankle, dknee, danke] = forward_kinimatics_leg(q,qd);
end

== matlab function Copy_of_sliding_controller/Enabled Subsystem3/F->tau1/Subsystem/MATLAB Function1 ==
  data: q input; y output
function y = fcn(q)

    l1 = 0.3240;
    l2 = 0.3900;
    y = [-l1*sin(q(1))-l2*sin(q(1)+q(2)), l1*cos(q(1)) + l2*sin(q(1)+q(2));...
         -l2*sin(q(1)+q(2)), l2*cos(q(1)+q(2))];
     
end

== matlab function Copy_of_sliding_controller/Enabled Subsystem3/F->tau/Subsystem2/MATLAB Function ==
  data: q input; y output
function y = fcn(q)

l1 = 0.3240;
y = [-l1*sin(q(1)), 0; l1*cos(q(1)), 0 ];


end

== matlab function Copy_of_sliding_controller/Enabled Subsystem3/F->tau/Subsystem2/MATLAB Function1 ==
  data: q input; y output
function y = fcn(q)

    l1 = 0.3240;
    l2 = 0.3900;
    y = [-l1*sin(q(1))-l2*sin(q(1)+q(2)), l1*cos(q(1)) + l2*sin(q(1)+q(2));...
         -l2*sin(q(1)+q(2)), l2*cos(q(1)+q(2))];
     
end

== matlab function Copy_of_sliding_controller/Enabled Subsystem3/F->tau1/Subsystem2/MATLAB Function ==
  data: q input; y output
function y = fcn(q)

l1 = 0.3240;
y = [-l1*sin(q(1)), 0; l1*cos(q(1)), 0 ];


end

== matlab function Copy_of_sliding_controller/Enabled Subsystem3/F->tau1/Subsystem2/MATLAB Function1 ==
  data: q input; y output
function y = fcn(q)

    l1 = 0.3240;
    l2 = 0.3900;
    y = [-l1*sin(q(1))-l2*sin(q(1)+q(2)), l1*cos(q(1)) + l2*sin(q(1)+q(2));...
         -l2*sin(q(1)+q(2)), l2*cos(q(1)+q(2))];
     
end

== matlab function Copy_of_sliding_controller/Enabled Subsystem3/sliding mode controller/MATLAB Function - String Array Assign ==
  data: blankMsg input; msg output Bus: SL_Bus_sliding_controller_RBDLInverseDynamicsReques_3qoi39
function msg = stringArrayAssign(blankMsg)
% stringArrayAssign - Assign a string array in a ROS message
%
%  blankMsg (input): A bus for a 'sensor_msgs/JointState' message. This is 
%      used to initialize the output.
%  msg (output): A bus for a 'sensor_msgs/JointState' message message, with 
%      Name field set to a string array.
%
%   Copyright 2015 The MathWorks, Inc.

%#codegen

% Note: The datatype of 'msg' has been explicitly set to the appropriate 
% Simulink bus type ("SL_Bus_robotROSMessageUsageExample_sensor_msgs_JointState"). 
%
% If the model name is changed, the datatype needs to be changed as well:
%   1) Click "Edit Data" in the Editor toolstrip to open "Ports and Data Manager"
%   2) Select "msg". From the "Type" dropdown, select "--- Refresh data types ---"
%   3) Set datatype to "Bus: SL_Bus_<modelname>_sensor_msgs_JointState"

strArrayToAssign = {'exo'};
msg = blankMsg;
name = 'exo';
strLength = length(name);
% Set the number of strings in the string array.
% msg (sensor_msgs/JointState) includes the following fields
%           Name : array of std_msgs/String (string array)
%   Name_SL_Info : struct with fields CurrentLength, ReceivedLength
numStringsInArray = length(strArrayToAssign);
%msg.ModelName.Data = uint8(name);
msg.ModelName_SL_Info.CurrentLength = uint32(strLength); % uint32(numStringsInArray);
msg.Q_SL_Info.CurrentLength = uint32(7);
msg.Qd_SL_Info.CurrentLength = uint32(7);
msg.Qdd_SL_Info.CurrentLength = uint32(7);

% % Set the individual strings in the array
% for idx=1:numStringsInArray
%     str = strArrayToAssign{idx};
%     strLength = length(str);
%     msg.ModelName(idx).Data(1:strLength) = uint8(str);
%     msg.Name(idx).Data_SL_Info.CurrentLength = uint32(strLength);
% end

== matlab function Copy_of_sliding_controller/Enabled Subsystem3/human controller/inv model 2/C ==
  data: m input; l input; q input; y output; qd input
function y = fcn(m, l, q, qd)



y = C(m, l, q, qd); % [m(2)*l(2)*qd(2)*qd(2)*sin(q(1)-q(2)); -m(2)*l(1)*qd(1)*qd(1)*sin(q(1)-q(2))];

== matlab function Copy_of_sliding_controller/Enabled Subsystem3/human controller/inv model 2/G ==
  data: m input; q input; y output
function y = fcn(m, q)
 y =  G(m,q);
end

== matlab function Copy_of_sliding_controller/Enabled Subsystem3/human controller/inv model 2/M ==
  data: m input; l input; q input; y output
function y = fcn(m, l, q)

y = M(m,l,q); % pinv([ (m(1)+m(2)) *l(1), m(2)*l(2)*cos(q(1)-q(2)); m(2)* l(1)*cos(q(1)-q(2)), m(2)*l(2)] );

end

== matlab function Copy_of_sliding_controller/Enabled Subsystem3/exo model/MATLAB Function - String Array Assign ==
  data: blankMsg input; msg output Bus: SL_Bus_sliding_controller_sensor_msgs_JointState
function msg = stringArrayAssign(blankMsg)
% stringArrayAssign - Assign a string array in a ROS message
%
%  blankMsg (input): A bus for a 'sensor_msgs/JointState' message. This is 
%      used to initialize the output.
%  msg (output): A bus for a 'sensor_msgs/JointState' message message, with 
%      Name field set to a string array.
%
%   Copyright 2015 The MathWorks, Inc.

%#codegen

% Note: The datatype of 'msg' has been explicitly set to the appropriate 
% Simulink bus type ("SL_Bus_robotROSMessageUsageExample_sensor_msgs_JointState"). 
%
% If the model name is changed, the datatype needs to be changed as well:
%   1) Click "Edit Data" in the Editor toolstrip to open "Ports and Data Manager"
%   2) Select "msg". From the "Type" dropdown, select "--- Refresh data types ---"
%   3) Set datatype to "Bus: SL_Bus_<modelname>_sensor_msgs_JointState"

strArrayToAssign = {'LeftExoHip', 'LeftExoKnee', 'LeftExoAnkle', 'RightExoHip', 'RightExoKnee', 'RightExoAnkle', 'Crutches'};
msg = blankMsg;

% Set the number of strings in the string array.
% msg (sensor_msgs/JointState) includes the following fields
%           Name : array of std_msgs/String (string array)
%   Name_SL_Info : struct with fields CurrentLength, ReceivedLength
numStringsInArray = length(strArrayToAssign);
msg.Name_SL_Info.CurrentLength = uint32(numStringsInArray);
msg.Effort_SL_Info.CurrentLength = uint32(numStringsInArray);

% Set the individual strings in the array
for idx=1:numStringsInArray
    str = strArrayToAssign{idx};
    strLength = length(str);
    msg.Name(idx).Data(1:strLength) = uint8(str);
    msg.Name(idx).Data_SL_Info.CurrentLength = uint32(strLength);
end

== matlab function Copy_of_sliding_controller/Enabled Subsystem3/ interaction sping-damper/human right ==
  data: q input; knee output; dknee output; qd input; ankle output; danke output
function [knee, dknee,ankle, danke]  = fcn(q, qd)


[knee, ankle, dknee, danke] = forward_kinimatics_leg(q,qd);
end

== matlab function Copy_of_sliding_controller/Enabled Subsystem3/F->tau/Subsystem/MATLAB Function ==
  data: q input; y output
function y = fcn(q)

l1 = 0.3240;
y = [-l1*sin(q(1)), 0; l1*cos(q(1)), 0 ];


end

== matlab function Copy_of_sliding_controller/Enabled Subsystem3/F->tau/Subsystem/MATLAB Function1 ==
  data: q input; y output
function y = fcn(q)

    l1 = 0.3240;
    l2 = 0.3900;
    y = [-l1*sin(q(1))-l2*sin(q(1)+q(2)), l1*cos(q(1)) + l2*sin(q(1)+q(2));...
         -l2*sin(q(1)+q(2)), l2*cos(q(1)+q(2))];
     
end

== matlab function Copy_of_sliding_controller/Enabled Subsystem3/addmittance1/MATLAB Function ==
  data: Tid input; K output; Th input; qd input; B output
function [K,B] = fcn(Tid, Th, qd)

Kp0 = 75*eye(7); %[75 0; 0 25];
Kn0 = 50*eye(7); %50*eye(7); % [50 0; 0 50];
Bp0 = 50*eye(7); %[75 0; 0 25];
Bn0 = 50*eye(7); %[50 0; 0 50];
beta_p = 3;
beta_n = 3;
alpha_p = 0.5;
alpha_n = 0.5;

intention = sign(Th) == sign(qd);
change = abs(Th/Tid);

K = eye(size(intention,1));
B = eye(size(intention,1));
count = 1;
my_intention = zeros(7,1);


for ii =  1:length(intention)
   if intention(ii)
        K(count,count) = Kp0(count,count) + beta_p*change(count);
        B(count,count) = Bp0(count,count) + alpha_p*change(count);
   else
       K(count,count) = Kn0(count,count) - beta_n*change(count);
       B(count,count) = Bn0(count,count) - alpha_n*change(count);
   end
   my_intention(count) = 0;
   count= count + 1;
   

end


end
